simulink model "Simulation"  (R2019a)
settings: Solver=VariableStepAuto  StartTime=0.0  StopTime=720  RelTol=1e-3
undefined symbols (not defined in the file or in its folder): m, n
libraries: Healthcare_Center_Department x1, Online_Application_Department x1
settings Model: Creator=arsineh  LastModifiedBy=arsineh

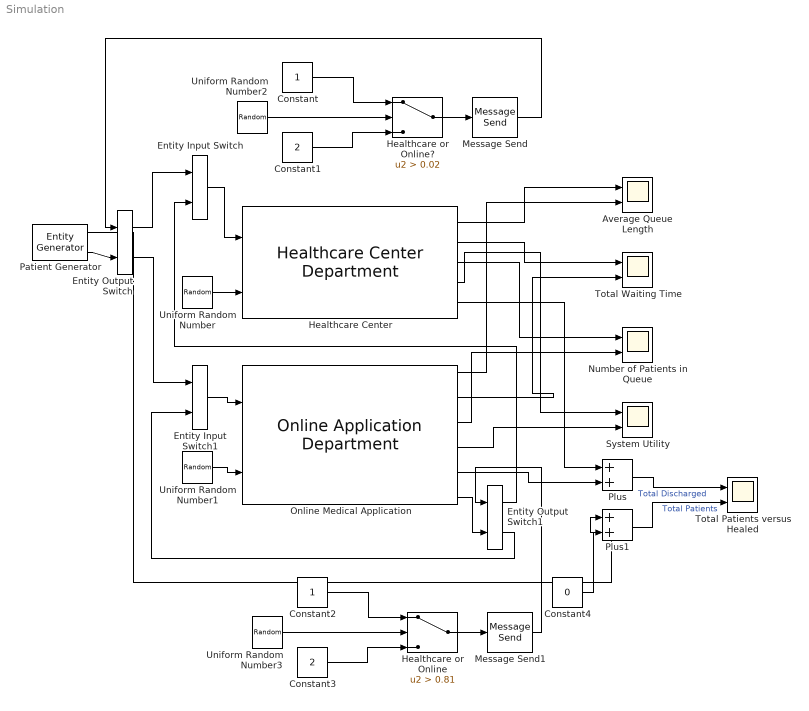
== system Simulation ==
  Average Queue Length : Scope  NumInputPorts=2
  Constant : Constant  VectorParams1D=off
  Constant1 : Constant  Value=2  VectorParams1D=off
  Constant2 : Constant  VectorParams1D=off
  Constant3 : Constant  Value=2  VectorParams1D=off
  Constant4 : Constant  Value=0
  Entity Input Switch : EntityInputSwitch  InputPortMessageModes=m,m  OutputPortMessageModes=m
  Entity Input Switch1 : EntityInputSwitch  InputPortMessageModes=m,m  OutputPortMessageModes=m
  Entity Output Switch : EntityOutputSwitch  InputPortMessageModes=m,m  OutputPortMessageModes=m,m  SwitchingCriterion=From control port  Seed=12345  SwitchAttributeName=Attribute1
      settings: InputPortMap=u0,u1
  Entity Output Switch1 : EntityOutputSwitch  InputPortMessageModes=m,m  OutputPortMessageModes=m,m  SwitchingCriterion=From control port  Seed=12345  SwitchAttributeName=Attribute1
      settings: InputPortMap=u0,u1
  Healthcare Center : Healthcare_Center_Department/Healthcare Center Department  SystemSampleTime=-1
  Healthcare or Online : Switch  Criteria=u2 > Threshold  Threshold=0.81
  Healthcare or Online? : Switch  Criteria=u2 > Threshold  Threshold=0.02
  Message Send : MessageSend  OutputPortMessageModes=m
      settings: InputPortMap=u1
  Message Send1 : MessageSend  OutputPortMessageModes=m
      settings: InputPortMap=u1
  Number of Patients in Queue : Scope  NumInputPorts=2
  Online Medical Application : Online_Application_Department/Online Application Department  SystemSampleTime=-1
  Patient Generator : EntityGenerator  OutputPortMessageModes=n,m  Period=0.00135  IntergenerationTimeAction=dt = randi([1,15]);  AttributeName=entity  AttributeInitialValue=0  NumberEntitiesDeparted=on  EntityTypeName=Entity
      settings: OutputPortMap=o0,o3
  Plus : Sum
  Plus1 : Sum
  System Utility : Scope  NumInputPorts=2
  Total Patients versus Healed : Scope  NumInputPorts=2
  Total Waiting Time : Scope  NumInputPorts=2
  Uniform Random Number : UniformRandomNumber  Minimum=3  Maximum=7.9  Seed=12345  SampleTime=0.01
  Uniform Random Number1 : UniformRandomNumber  Minimum=1  Maximum=3  Seed=12345  SampleTime=0.01
  Uniform Random Number2 : UniformRandomNumber  Minimum=0  Seed=1325435  SampleTime=0.01
  Uniform Random Number3 : UniformRandomNumber  Minimum=0  Seed=1325435  SampleTime=0.01
  wires:
  Patient Generator/2 -> Entity Output Switch/2
  Uniform Random Number/1 -> Healthcare Center/2
  Uniform Random Number1/1 -> Online Medical Application/2
  Healthcare Center/1 -> Average Queue Length/1
  Online Medical Application/2 -> Total Waiting Time/2
  Online Medical Application/1 -> Average Queue Length/2
  Entity Output Switch/2 -> Entity Input Switch1/1
  Entity Output Switch1/1 -> Entity Input Switch/2
  Entity Output Switch/1 -> Entity Input Switch/1
  Entity Input Switch/1 -> Healthcare Center/1
  Healthcare Center/2 -> Total Waiting Time/1
  Constant/1 -> Healthcare or Online?/1
  Uniform Random Number2/1 -> Healthcare or Online?/2
  Healthcare or Online?/1 -> Message Send/1
  Constant1/1 -> Healthcare or Online?/3
  Message Send/1 -> Entity Output Switch/1
  Online Medical Application/6 -> Entity Output Switch1/2
  Message Send1/1 -> Entity Output Switch1/1
  Constant3/1 -> Healthcare or Online/3
  Healthcare or Online/1 -> Message Send1/1
  Uniform Random Number3/1 -> Healthcare or Online/2
  Constant2/1 -> Healthcare or Online/1
  Entity Output Switch1/2 -> Entity Input Switch1/2
  Entity Input Switch1/1 -> Online Medical Application/1
  Healthcare Center/3 -> Number of Patients in Queue/1
  Online Medical Application/3 -> Number of Patients in Queue/2
  Healthcare Center/4 -> System Utility/1
  Online Medical Application/4 -> System Utility/2
  Healthcare Center/5 -> Plus/1
  Online Medical Application/5 -> Plus/2
  Plus/1 -> Total Patients versus Healed/1  "Total Discharged"
  Patient Generator/1 -> Plus1/1
  Constant4/1 -> Plus1/2
  Plus1/1 -> Total Patients versus Healed/2  "Total Patients"
